simulink model "ASM_Traffic_V2X_Complete_Model_2"  (R2019a)
settings: Solver=ode1  StartTime=SIM.tstart.v  StopTime=Inf  FixedStep=SIM.StepSize.v  RelTol=1e-3
PostLoadFcn:
  | if any(exist('dsrtsu_mdlpostloadfcn', 'file') ~= 0), dsrtsu_mdlpostloadfcn('Execute', bdroot); end
  | try, asm_mdl_postloadfcn(bdroot, 'UpdateModel', 2200); catch, disp(lasterr); end,
undefined symbols (not defined in the file): _SensorPnts_1, _SensorPnts_13, _SensorPnts_17, _SensorPnts_21, _SensorPnts_25, _SensorPnts_29, _SensorPnts_33, _SensorPnts_37, _SensorPnts_41, _SensorPnts_45, _SensorPnts_49, _SensorPnts_5, _SensorPnts_53, _SensorPnts_57, _SensorPnts_9, _to_, CPT, G5A, ITS, MDL, rad, s_to_rpm, SIM
libraries: simulink x169, ASM_VehicleDynamics_lib x126, ASM_Traffic_lib x83, ASM_Utils_lib x49, mdbs x45, ASM_Environment_lib x17, dspindex x12, dsaV2xLibraryAux x10, dsmpblib x6, dsaV2xAsn1Library x4, dsaV2xLibrary x4, ASM_BrakeHydraulics_lib x4
(part 3 of 36)

== system ASM_Traffic_V2X_Complete_Model_2/IO/I//O_Subsystem/EgoCar_Command ==
  In1 : Inport
  In2 : Inport  Port=2
  Bus Creator : BusCreator  Inputs=4
  Bus Selector : BusSelector  OutputSignals=Simulated ECUs.DrivekitCAN.Drivekit.RX.PDUs.THROTTLE_COMMAND.throttle_pedal_command.ISignal Value.throttle_pedal_command Value,Simulated ECUs.DrivekitCAN.Drivekit.RX.PDUs.BRAKE_COMMAND.brake_pedal_command.ISignal Value.brake_pedal_command Value,Simulated ECUs.DrivekitCAN.Drivekit.RX.PDUs.STEERING_ANGLE_COMMAND.steering_angle_cmd_angle.ISignal Value.steering_angle_cmd_angle Value
  Data Type Conversion : DataTypeConversion  OutDataTypeStr=double
  Data Type Conversion1 : DataTypeConversion  OutDataTypeStr=double
  Data Type Conversion2 : DataTypeConversion  OutDataTypeStr=double
  Gain : Gain  Gain=100
  Gain1 : Gain  Gain=100
  Out1 : Outport
  wires:
  Gain1/1 -> Bus Creator/2
  Data Type Conversion1/1 -> Gain1/1
  Gain/1 -> Bus Creator/1
  Data Type Conversion/1 -> Gain/1
  Bus Creator/1 -> Out1/1
  In2/1 -> Bus Creator/4
  In1/1 -> Bus Selector/1
  Data Type Conversion2/1 -> Bus Creator/3
  Bus Selector/2 -> Data Type Conversion1/1  "<brake_pedal_command Value>"
  Bus Selector/3 -> Data Type Conversion2/1  "<steering_angle_cmd_angle Value>"
  Bus Selector/1 -> Data Type Conversion/1  "<throttle_pedal_command Value>"

== system ASM_Traffic_V2X_Complete_Model_2/IO/I//O_Subsystem/EgoCar_Data ==
  In1 : Inport
  Bus Creator : BusCreator  Inputs=4
  GPS : Subsystem
  Lane_Number : Subsystem
  Steering_Angle : Subsystem
  Wheel_Speed : Subsystem
  Out1 : Outport
  wires:
  Bus Creator/1 -> Out1/1
  GPS/1(Out1) -> Bus Creator/3
  Wheel_Speed/1(Out1) -> Bus Creator/2
  Steering_Angle/1(Out1) -> Bus Creator/1
  In1/1 -> Steering_Angle/1(In1), Wheel_Speed/1(In1), Lane_Number/1(In1), GPS/1(In1)
  Lane_Number/1(Out1) -> Bus Creator/4

== system ASM_Traffic_V2X_Complete_Model_2/IO/V2X_Subsystem/CAM-DENM_Message_Generation ==
  note: DENM
  note: CAM
  Input : Inport
  Bus Selector : BusSelector  OutputSignals=signal1,signal2,signal3,GenDENMData
  DENM : Subsystem
  Fellow_CAM_1 : Subsystem
  Fellow_CAM_2 : Subsystem
  Fellow_CAM_3 : Subsystem
  MSG_FREQ : DiscretePulseGenerator  PulseType=Time based  Period=0.5  PulseWidth=90
  Mux2 : Mux  Inputs=2
  Mux3 : Mux  Inputs=2
  Mux5 : Mux  Inputs=2
  OR : Logic  Operator=OR  Inputs=3  IconShape=distinctive  AllPortsSameDT=off  OutDataTypeStr=boolean
  Queue_CAM : Subsystem  TreatAsAtomicUnit=on
  Queue_CAM_DENM : Subsystem  TreatAsAtomicUnit=on
  Send_UDP : Subsystem  TreatAsAtomicUnit=on
  V2X_FREQ : DiscretePulseGenerator  PulseType=Time based  Period=0.5  PulseWidth=90
  wires:
  Queue_CAM_DENM/1(Data) -> Send_UDP/1(In1)
  V2X_FREQ/1 -> Send_UDP/Trigger
  MSG_FREQ/1 -> Queue_CAM_DENM/Trigger
  Queue_CAM_DENM/2(Byte) -> Send_UDP/2(Input)
  Mux5/1 -> Queue_CAM/1(Fellow_1)
  Fellow_CAM_2/1(Data) -> Mux3/1
  Fellow_CAM_2/2(Bytes) -> Mux3/2
  Fellow_CAM_1/1(Data) -> Mux5/1
  Fellow_CAM_1/2(Bytes) -> Mux5/2
  Mux2/1 -> Queue_CAM/3(Fellow_3)
  Fellow_CAM_3/1(Data) -> Mux2/1
  Fellow_CAM_3/2(Bytes) -> Mux2/2
  Mux3/1 -> Queue_CAM/2(Fellow_2)
  Fellow_CAM_1/3(Output_Enabler) -> OR/1, Queue_CAM/4(Enable_CAM1)
  Fellow_CAM_2/3(Output_Enabler) -> OR/2, Queue_CAM/5(Enable_CAM2)
  Fellow_CAM_3/3(Output_Enabler) -> OR/3, Queue_CAM/6(Enable_CAM3)
  OR/1 -> Queue_CAM_DENM/3(Enable_CAM), Queue_CAM/Enable
  Queue_CAM/1(OutputCAM) -> Queue_CAM_DENM/1(cam)
  DENM/1(denm_freq) -> Queue_CAM_DENM/4(Enable_DENM)
  DENM/2(denm) -> Queue_CAM_DENM/2(denm)
  Input/1 -> Bus Selector/1
  Bus Selector/1 -> Fellow_CAM_1/1(Input)  "<signal1>"
  Bus Selector/2 -> Fellow_CAM_2/1(Input)  "<signal2>"
  Bus Selector/3 -> Fellow_CAM_3/1(Input)  "<signal3>"
  Bus Selector/4 -> DENM/1("GENDENMData ")  "<GenDENMData>"

== system ASM_Traffic_V2X_Complete_Model_2/IO/V2X_Subsystem/Car_Data ==
  Fellow_Pos_info : Inport
  Bus Creator : BusCreator  Inputs=4
  EGOCAR_Position : Subsystem
  Fellow_ID_1 : Subsystem
  Fellow_ID_2 : Subsystem
  Fellow_ID_3 : Subsystem
  Subsystem : Subsystem
  Output : Outport
  wires:
  Bus Creator/1 -> Output/1
  Fellow_ID_3/1(Output) -> Bus Creator/3
  Fellow_ID_2/1(Output) -> Bus Creator/2
  Fellow_ID_1/1(Output) -> Bus Creator/1
  EGOCAR_Position/1(Output) -> Fellow_ID_1/1("EGO_Car_Position "), Subsystem/2(Input), Fellow_ID_3/1("EGO_Car_Position "), Fellow_ID_2/1("EGO_Car_Position ")
  Fellow_Pos_info/1 -> Fellow_ID_1/2(Input), Subsystem/3(Input1), Subsystem/1(In1), Fellow_ID_3/2(Input), Fellow_ID_2/2(Input), EGOCAR_Position/1(In1)
  Subsystem/1(Out1) -> Bus Creator/4

== system ASM_Traffic_V2X_Complete_Model_2/IO/V2X_Subsystem/Subsystem ==
  In1 : Inport
  AND : Logic  IconShape=distinctive  AllPortsSameDT=off  OutDataTypeStr=boolean
  AND1 : Logic  IconShape=distinctive  AllPortsSameDT=off  OutDataTypeStr=boolean
  AND_Display : Display
  Bus Selector : BusSelector  OutputSignals=Environment.Maneuver.ManeuverScheduler.Info.s_local[m],Environment.Maneuver.ManeuverScheduler.Info.t_local[s],Environment.Maneuver.ManeuverScheduler.Info.ManeuverTime[s],Environment.Driver.OutputSignals.Pos_BrakePedal[%],VehicleDynamics.VehicleMovement.Velocities.Vehicle.Linear.v_Vehicle_CoG[x;y;z][km|h].v_x_Vehicle_CoG[km|h],VehicleDynamics.VehicleMovement.Velocities.Vehicle.Linear.v_Total_Vehicle[km|h]
  Constant : Constant  Value=20
  Constant1 : Constant  Value=20
  Constant2 : Constant  Value=19.8
  Data Type Conversion{,1..4} (5 alike) : DataTypeConversion
  Relational Operator : RelationalOperator  Operator=<=  OutDataTypeStr=boolean  RndMeth=Simplest
  Relational Operator1 : RelationalOperator  OutDataTypeStr=boolean  RndMeth=Simplest
  Relational Operator2 : RelationalOperator  OutDataTypeStr=boolean  RndMeth=Simplest
  Subsystem : Subsystem
  driven_distance : Display
  manuever_time : Display
  pos_brake_pedal : Display
  speed_disp : Display
  start_of_spot_search : Display
  t_local : Display
  time_disp : Display
  v_ttotal_vehicle : Display
  v_x_vehicle : Display
  wires:
  In1/1 -> Bus Selector/1
  Bus Selector/1 -> Subsystem/1(In1), driven_distance/1  "<s_local[m]>"
  Bus Selector/2 -> t_local/1  "<t_local[s]>"
  Bus Selector/3 -> Relational Operator1/1, manuever_time/1  "<ManeuverTime[s]>"
  Bus Selector/4 -> pos_brake_pedal/1  "<Pos_BrakePedal[%]>"
  Bus Selector/5 -> Relational Operator2/1, Relational Operator/1, v_x_vehicle/1  "<v_x_Vehicle_CoG[km|h]>"
  Bus Selector/6 -> v_ttotal_vehicle/1  "<v_Total_Vehicle[km|h]>"
  Constant/1 -> Relational Operator/2
  Constant1/1 -> Relational Operator1/2
  Relational Operator1/1 -> Data Type Conversion/1
  Subsystem/1(Output) -> start_of_spot_search/1
  Constant2/1 -> Relational Operator2/2
  Relational Operator/1 -> Data Type Conversion1/1
  Relational Operator2/1 -> Data Type Conversion4/1
  AND1/1 -> Data Type Conversion2/1
  Data Type Conversion/1 -> time_disp/1, AND/1
  Data Type Conversion1/1 -> AND1/1, speed_disp/1
  Data Type Conversion2/1 -> AND/2
  AND/1 -> Data Type Conversion3/1
  Data Type Conversion3/1 -> Subsystem/Trigger, AND_Display/1
  Data Type Conversion4/1 -> AND1/2

== system ASM_Traffic_V2X_Complete_Model_2/MDL/Drivetrain/ASMSignalCollector ==
  BusCreator : BusCreator  Inputs=5
  tag scope: ASMBUS_Drivetrain=global
  wires:
  [ASMBUS_Drivetrain_FinalDriveAssembly] -> BusCreator/2
  [ASMBUS_Drivetrain_Test_Bench] -> BusCreator/5
  [ASMBUS_Drivetrain_Starter] -> BusCreator/4
  [ASMBUS_Drivetrain_CrankShaft] -> BusCreator/3
  [ASMBUS_Transmission] -> BusCreator/1
  BusCreator/1 -> [ASMBUS_Drivetrain]  "Drivetrain"

== system ASM_Traffic_V2X_Complete_Model_2/MDL/Drivetrain/Crankshaft ==
  Trq_TestBench[Nm] : Inport
  Trq_External[Nm] : Inport  Port=2
  Inertia_External[kgm2] : Inport  Port=3
  Reset[0|1] : Inport  Port=4
  Trq_Engine[Nm] : Inport  Port=5
  Trq_Fric_Clutch[Nm] : Inport  Port=6
  CRANK_SHAFT : ASM_VehicleDynamics_lib/Drivetrain/Crankshaft_and_Starter/CRANK_SHAFT  Tag=ASM_SUBCOMPONENT  Const_Inertia=MDL.Drivetrain.CrankShaft.Const_Inertia  Map_Trq_Mass=MDL.Drivetrain.CrankShaft.Map_Trq_Mass_Mod  Sw_Trq_Mass_Mode=MDL.Drivetrain.CrankShaft.Sw_Trq_Mass_Mode  StepSize=SIM.StepSize  ASMProperties=struct('Name','CRANK_SHAFT','Version','9.0','Library','ASM_VehicleDynamics_lib')  ASMInstanceName=crank_shaft  ASMInstanceID=1
  CrankAngle_Cyl[deg] : Constant  Value=0
  FROM_STABILIZATION_CRANK_SHAFT : ASM_VehicleDynamics_lib/Drivetrain/Stabilization/FROM_STABILIZATION  Tag=ASM_SUBCOMPONENT  Stabi_Block=CRANK_SHAFT  Stabi_Block_ID=1  ASMProperties=struct('Name','FROM_STABILIZATION','Version','1.0','Library','ASM_VehicleDynamics_lib')  ASMInstanceName=from_stabilization  ASMInstanceID=1
      settings: AttributesFormatString=Destination: CRANK_SHAFT_ID1
  TO_STABILIZATION_CRANK_SHAFT : ASM_VehicleDynamics_lib/Drivetrain/Stabilization/TO_STABILIZATION  Tag=ASM_SUBCOMPONENT  Stabi_Block=CRANK_SHAFT  Stabi_Block_ID=1  ASMProperties=struct('Name','TO_STABILIZATION','Version','1.0','Library','ASM_VehicleDynamics_lib')  ASMInstanceName=to_stabilization  ASMInstanceID=1
      settings: AttributesFormatString=Source: CRANK_SHAFT_ID1
  n_Engine_Init[rad|s] : Constant  Value=0
  n_Engine[rpm] : Outport
  n_Engine[rad|s] : Outport  Port=2
  tag scope: ASMBUS_Drivetrain_CrankShaft=global
  wires:
  FROM_STABILIZATION_CRANK_SHAFT/1 -> CRANK_SHAFT/9
  Trq_Fric_Clutch[Nm]/1 -> CRANK_SHAFT/3
  Inertia_External[kgm2]/1 -> CRANK_SHAFT/5
  Trq_TestBench[Nm]/1 -> CRANK_SHAFT/6
  Reset[0|1]/1 -> CRANK_SHAFT/4
  n_Engine_Init[rad|s]/1 -> CRANK_SHAFT/8
  CrankAngle_Cyl[deg]/1 -> CRANK_SHAFT/7
  Trq_Engine[Nm]/1 -> CRANK_SHAFT/2
  Trq_External[Nm]/1 -> CRANK_SHAFT/1
  CRANK_SHAFT/4 -> TO_STABILIZATION_CRANK_SHAFT/1
  CRANK_SHAFT/3 -> n_Engine[rad|s]/1
  CRANK_SHAFT/2 -> n_Engine[rpm]/1
  CRANK_SHAFT/1 -> [ASMBUS_Drivetrain_CrankShaft]

== system ASM_Traffic_V2X_Complete_Model_2/MDL/Drivetrain/DisableReset ==
  Reset_VehicleStates[0|1] : Inport
  MultiPortSwitch : MultiPortSwitch  DataPortOrder=Zero-based contiguous  Inputs=2  zeroidx=on  SaturateOnIntegerOverflow=on  InputSameDT=on
  NO_Reset : Constant  Value=0
  Reset[0|1] : Outport
  wires:
  Reset_VehicleStates[0|1]/1 -> MultiPortSwitch/3
  NO_Reset/1 -> MultiPortSwitch/2
  [TAG_Drivetrain_Sw_CrankShaft_Reset] -> MultiPortSwitch/1
  MultiPortSwitch/1 -> Reset[0|1]/1

== system ASM_Traffic_V2X_Complete_Model_2/MDL/Drivetrain/External Loads ==
  Inertia_TestBench[kgm2] : Inport
  Trq_Starter[Nm] : Inport  Port=2
  Inertia_Starter[kgm2] : Inport  Port=3
  Sw_AC[0|1] : Inport  Port=4
  Intertia_AC[kgm2] : Gain  Gain=0  SaturateOnIntegerOverflow=on  OutDataTypeStr=Inherit: Same as input  ParamDataTypeStr=Inherit: Same as input
  ManualLoadTorque : Subsystem
  Sum : Sum  Inputs=+++  SaturateOnIntegerOverflow=on
  Sum1 : Sum  Inputs=-+|  SaturateOnIntegerOverflow=on
  Trq_AC[Nm] : Gain  Gain=0  SaturateOnIntegerOverflow=on  OutDataTypeStr=Inherit: Same as input  ParamDataTypeStr=Inherit: Same as input
  Trq_External[Nm] : Outport
  Intertia_External[kgm2] : Outport  Port=2
  wires:
  Inertia_TestBench[kgm2]/1 -> Sum/1
  Intertia_AC[kgm2]/1 -> Sum/3
  Inertia_Starter[kgm2]/1 -> Sum/2
  ManualLoadTorque/1(Out) -> Trq_External[Nm]/1
  Trq_AC[Nm]/1 -> Sum1/1
  Sum1/1 -> ManualLoadTorque/1(In)
  Trq_Starter[Nm]/1 -> Sum1/2
  Sw_AC[0|1]/1 -> Trq_AC[Nm]/1, Intertia_AC[kgm2]/1
  Sum/1 -> Intertia_External[kgm2]/1

== system ASM_Traffic_V2X_Complete_Model_2/MDL/Drivetrain/Final_Drive_Assembly ==
  Inertia_Trm[kgm2] : Inport
  Trq_Out_Trm[Nm] : Inport  Port=2
  Reset[0|1] : Inport  Port=3
  omega_Wheel[FL,FR,RL,RR][rad|s] : Inport  Port=4
  ASMSignalCollector : Subsystem
  Differentials : Subsystem
  FF4WD_Parts : Subsystem
  GotoTagVisibility_CentralDifferential : GotoTagVisibility  GotoTag=ASMBUS_Drivetrain_CentralDifferential
  GotoTagVisibility_Clutch_4WD : GotoTagVisibility  GotoTag=ASMBUS_Drivetrain_Clutch_4WD
  GotoTagVisibility_FrontDifferential : GotoTagVisibility  GotoTag=ASMBUS_Drivetrain_FrontDifferential
  GotoTagVisibility_RearDifferential : GotoTagVisibility  GotoTag=ASMBUS_Drivetrain_RearDifferential
  GotoTagVisibility_Shaft_CF : GotoTagVisibility  GotoTag=ASMBUS_Drivetrain_Shaft_CF
  GotoTagVisibility_Shaft_CR : GotoTagVisibility  GotoTag=ASMBUS_Drivetrain_Shaft_CR
  GotoTagVisibility_Shaft_FL : GotoTagVisibility  GotoTag=ASMBUS_Drivetrain_Shaft_FL
  GotoTagVisibility_Shaft_FR : GotoTagVisibility  GotoTag=ASMBUS_Drivetrain_Shaft_FR
  GotoTagVisibility_Shaft_RL : GotoTagVisibility  GotoTag=ASMBUS_Drivetrain_Shaft_RL
  GotoTagVisibility_Shaft_RR : GotoTagVisibility  GotoTag=ASMBUS_Drivetrain_Shaft_RR
  GotoTagVisibility_Shaft_TGCL4WD : GotoTagVisibility  GotoTag=ASMBUS_Drivetrain_Shaft_TGCL4WD
  GotoTagVisibility_Transfer_Gearbox : GotoTagVisibility  GotoTag=ASMBUS_Drivetrain_Transfer_Gearbox
  STABILIZATION : Subsystem
  Shafts : Subsystem
  SignalSelection : Subsystem
  omega_In_Diff[rad|s] : Outport
  Trq_Shaft[FL,FR,RL,RR][Nm] : Outport  Port=2
  wires:
  Reset[0|1]/1 -> FF4WD_Parts/3(Reset[0|1]), Shafts/10(Reset[0|1]), Differentials/15(Reset[0|1])
  FF4WD_Parts/1(Inertia_Out_Clutch4WD[kgm2]) -> SignalSelection/6(Inertia_Out_Clutch4WD[kgm2])
  FF4WD_Parts/2(Trq_Lock_Clutch4WD[Nm]) -> SignalSelection/5(Trq_Lock_Clutch4WD[Nm])
  FF4WD_Parts/3(Inertia_In_TransferGearbox[kgm2]) -> SignalSelection/4(Inertia_In_TransferGearbox[kgm2])
  FF4WD_Parts/4(Trq_In_TransferGearbox[Nm]) -> SignalSelection/3(Trq_In_TransferGearbox[Nm])
  SignalSelection/6(Inertia_External_InputShaft_RearDiff[kgm2]) -> Differentials/8(Inertia_External_InputShaft_RearDiff[kgm2])
  SignalSelection/5(Trq_In_RearDiff[Nm]) -> Differentials/7(Trq_In_RearDiff[Nm])
  SignalSelection/4(Inertia_Ext_Cage_FrontDiff[kgm2]) -> Differentials/6(Inertia_Ext_Cage_FrontDiff[kgm2])
  SignalSelection/3(Trq_Ext_Cage_FrontDiff[Nm]) -> Differentials/5(Trq_Ext_Cage_FrontDiff[Nm])
  SignalSelection/2(Inertia_External_InputShaft_FrontDiff[kgm2]) -> Differentials/4(Inertia_External_InputShaft_FrontDiff[kgm2])
  SignalSelection/1(Trq_In_FrontDiff[Nm]) -> Differentials/3(Trq_In_FrontDiff[Nm])
  Differentials/2(omega_Cage_FrontDiff[rad|s]) -> FF4WD_Parts/5(omega_Cage_FrontDiff[rad|s])
  Differentials/3(omega_In_RearDiff[rad|s]) -> FF4WD_Parts/4(omega_In_RearDiff[rad|s]), Shafts/8(omega_In_RearDiff[rad|s])
  Differentials/4(omega_In_FrontDiff[rad|s]) -> Shafts/7(omega_In_FrontDiff[rad|s])
  Differentials/6(omega_Out_Rear_CentralDiff[rad|s]) -> Shafts/5(omega_Out_Rear_CentralDiff[rad|s])
  Differentials/5(omega_Out_Front_CentralDiff[rad|s]) -> Shafts/6(omega_Out_Front_CentralDiff[rad|s])
  Shafts/4(Trq_CR_Shaft[Nm]) -> Differentials/11(Trq_CR_Shaft[Nm]), SignalSelection/8(Trq_CR_Shaft[Nm])
  Shafts/3(Trq_CF_Shaft[Nm]) -> Differentials/12(Trq_CF_Shaft[Nm]), SignalSelection/7(Trq_CF_Shaft[Nm])
  omega_Wheel[FL,FR,RL,RR][rad|s]/1 -> Shafts/9(omega_Wheel[FL,FR,RL,RR][rad|s])
  Shafts/7(Trq_Shaft[FL,FR,RL,RR][Nm]) -> Trq_Shaft[FL,FR,RL,RR][Nm]/1
  Differentials/10(omega_Out_Right_RearDiff[rad|s]) -> Shafts/1(omega_Out_Right_RearDiff[rad|s])
  Differentials/9(omega_Out_Left_RearDiff[rad|s]) -> Shafts/2(omega_Out_Left_RearDiff[rad|s])
  Differentials/8(omega_Out_Right_FrontDiff[rad|s]) -> Shafts/3(omega_Out_Right_FrontDiff[rad|s])
  Differentials/7(omega_Out_Left_FrontDiff[rad|s]) -> Shafts/4(omega_Out_Left_FrontDiff[rad|s])
  Differentials/1(omega_In_Diff[rad|s]) -> omega_In_Diff[rad|s]/1
  Shafts/5(Trq_RR_Shaft[Nm]) -> FF4WD_Parts/2(Trq_RR_Shaft[Nm]), Differentials/10(Trq_RR_Shaft[Nm])
  Shafts/6(Trq_RL_Shaft[Nm]) -> FF4WD_Parts/1(Trq_RL_Shaft[Nm]), Differentials/9(Trq_RL_Shaft[Nm])
  Shafts/1(Trq_FR_Shaft[Nm]) -> Differentials/14(Trq_FR_Shaft[Nm])
  Shafts/2(Trq_FL_Shaft[Nm]) -> Differentials/13(Trq_FL_Shaft[Nm])
  Trq_Out_Trm[Nm]/1 -> Differentials/2(Trq_Out_Trm[Nm]), SignalSelection/2(Trq_Out_Trm[Nm])
  Inertia_Trm[kgm2]/1 -> Differentials/1(Inertia_Trm[kgm2]), SignalSelection/1(Inertia_Trm[kgm2])

== system ASM_Traffic_V2X_Complete_Model_2/MDL/Drivetrain/OpenCrankshaftDemos ==

== system ASM_Traffic_V2X_Complete_Model_2/MDL/Drivetrain/OpenFinalDriveAssemblyDemos ==

== system ASM_Traffic_V2X_Complete_Model_2/MDL/Drivetrain/OpenTransmissionSystemDemos ==

== system ASM_Traffic_V2X_Complete_Model_2/MDL/Drivetrain/Transmission ==
  Trq_Engine[Nm] : Inport
  n_Engine[rad|s] : Inport  Port=2
  Ctrl_Lockup_Clutch[%] : Inport  Port=3
  Gear_AT[] : Inport  Port=4
  Pos_ClutchPedal_MT[%] : Inport  Port=5
  Gear_MT[] : Inport  Port=6
  SW_TrmMode[1Manual|2Automatic] : Inport  Port=7
  Reset[0|1] : Inport  Port=8
  omega_In_Diff[rad|s] : Inport  Port=9
  ASMSignalCollector : Subsystem
  AutomaticActive : simulink/Logic and Bit Operations/Compare To Constant  relop===  const=2  OutDataTypeStr=boolean
  AutomaticTransmission : Subsystem  TreatAsAtomicUnit=on
  FROM_STABILIZATION_CLUTCH : ASM_VehicleDynamics_lib/Drivetrain/Stabilization/FROM_STABILIZATION  Tag=ASM_SUBCOMPONENT  Stabi_Block=CLUTCH  Stabi_Block_ID=1  ASMProperties=struct('Name','FROM_STABILIZATION','Version','1.0','Library','ASM_VehicleDynamics_lib')  ASMInstanceName=from_stabilization  ASMInstanceID=1
      settings: AttributesFormatString=Destination: CLUTCH_ID1
  ManualActive : simulink/Logic and Bit Operations/Compare To Constant  relop===  const=1  OutDataTypeStr=boolean
  ManualTransmission : Subsystem  TreatAsAtomicUnit=on
  Multiport Switch{,1..5} (6 alike) : MultiPortSwitch  Inputs=2  SaturateOnIntegerOverflow=on
  Sat_TrmMode : Saturate  UpperLimit=2  LowerLimit=1
  TO_STABILIZATION_CLUTCH : ASM_VehicleDynamics_lib/Drivetrain/Stabilization/TO_STABILIZATION  Tag=ASM_SUBCOMPONENT  Stabi_Block=CLUTCH  Stabi_Block_ID=1  ASMProperties=struct('Name','TO_STABILIZATION','Version','1.0','Library','ASM_VehicleDynamics_lib')  ASMInstanceName=to_stabilization  ASMInstanceID=1
      settings: AttributesFormatString=Source: CLUTCH_ID1
  TO_STABILIZATION_GEARBOX : ASM_VehicleDynamics_lib/Drivetrain/Stabilization/TO_STABILIZATION  Tag=ASM_SUBCOMPONENT  Stabi_Block=GEARBOX  Stabi_Block_ID=1  ASMProperties=struct('Name','TO_STABILIZATION','Version','1.0','Library','ASM_VehicleDynamics_lib')  ASMInstanceName=to_stabilization  ASMInstanceID=1
      settings: AttributesFormatString=Source: GEARBOX_ID1
  TO_STABILIZATION_TORQUE_CONVERTER : ASM_VehicleDynamics_lib/Drivetrain/Stabilization/TO_STABILIZATION  Tag=ASM_SUBCOMPONENT  Stabi_Block=TORQUE_CONVERTER  Stabi_Block_ID=1  ASMProperties=struct('Name','TO_STABILIZATION','Version','1.0','Library','ASM_VehicleDynamics_lib')  ASMInstanceName=to_stabilization  ASMInstanceID=1
      settings: AttributesFormatString=Source: TORQUE_CONVERTER_ID1
  Trq_Fric[Nm] : Outport
  Inertia_Out_Trm[kgm2] : Outport  Port=2
  Trq_Out_Trm[Nm] : Outport  Port=3
  tag scope: ASMBUS_Drivetrain_AutomaticTransmission=global, ASMBUS_Drivetrain_ManualTransmission=global
  wires:
  Multiport Switch5/1 -> TO_STABILIZATION_CLUTCH/1
  Multiport Switch4/1 -> TO_STABILIZATION_GEARBOX/1
  ManualTransmission/5(TO_STABILIZATION_GEARBOX) -> Multiport Switch4/2
  AutomaticTransmission/6(TO_STABILIZATION_CLUTCH) -> Multiport Switch5/3
  AutomaticTransmission/7(TO_STABILIZATION_TORQUE_CONVERTER) -> TO_STABILIZATION_TORQUE_CONVERTER/1
  Sat_TrmMode/1 -> Multiport Switch/1, Multiport Switch1/1, Multiport Switch2/1, Multiport Switch4/1, Multiport Switch5/1, ASMSignalCollector/1(SW_TrmMode[]), Multiport Switch3/1, ManualActive/1, AutomaticActive/1
  Reset[0|1]/1 -> AutomaticTransmission/7(Reset[0|1]), ManualTransmission/7(Reset[0|1])
  AutomaticTransmission/5(TO_STABILIZATION_GEARBOX) -> Multiport Switch4/3
  AutomaticTransmission/4(Inertia_Out_Trm[kgm2]) -> Multiport Switch2/3
  AutomaticTransmission/3(Trq_Out_Trm[Nm]) -> Multiport Switch1/3
  AutomaticTransmission/2(Trq_In_Converter[Nm]) -> Multiport Switch/3
  ManualTransmission/6(TO_STABILIZATION_CLUTCH) -> Multiport Switch5/2
  Multiport Switch1/1 -> Trq_Out_Trm[Nm]/1
  Multiport Switch/1 -> Trq_Fric[Nm]/1
  Multiport Switch2/1 -> Inertia_Out_Trm[kgm2]/1
  ManualTransmission/2(Trq_Fric[Nm]) -> Multiport Switch/2
  ManualTransmission/3(Trq_Out_Trm[Nm]) -> Multiport Switch1/2
  ManualTransmission/4(Inertia_Out_Trm[kgm2]) -> Multiport Switch2/2
  SW_TrmMode[1Manual|2Automatic]/1 -> Sat_TrmMode/1
  Pos_ClutchPedal_MT[%]/1 -> ManualTransmission/1(Pos_Clutch[%])
  Gear_MT[]/1 -> ManualTransmission/2(Gear[]), Multiport Switch3/2
  n_Engine[rad|s]/1 -> AutomaticTransmission/3(n_Engine[rad|s]), ManualTransmission/3(n_Engine[rad|s])
  Trq_Engine[Nm]/1 -> AutomaticTransmission/4(Trq_Engine[Nm]), ManualTransmission/4(Trq_Engine[Nm])
  omega_In_Diff[rad|s]/1 -> AutomaticTransmission/5(omega_In_Diff[rad|s]), ManualTransmission/5(omega_In_Diff[rad|s])
  AutomaticActive/1 -> AutomaticTransmission/Enable
  FROM_STABILIZATION_CLUTCH/1 -> AutomaticTransmission/6(FROM_STABILIZATION_CLUTCH), ManualTransmission/6(FROM_STABILIZATION_CLUTCH)
  ManualActive/1 -> ManualTransmission/Enable
  Ctrl_Lockup_Clutch[%]/1 -> AutomaticTransmission/1(Ctrl_Lockup_Clutch[%])
  Gear_AT[]/1 -> AutomaticTransmission/2(Gear[]), Multiport Switch3/3
  Multiport Switch3/1 -> ASMSignalCollector/2(Gear[])
  ManualTransmission/1(ASMSignalBus) -> [ASMBUS_Drivetrain_ManualTransmission]
  AutomaticTransmission/1(ASMSignalBus) -> [ASMBUS_Drivetrain_AutomaticTransmission]

== system ASM_Traffic_V2X_Complete_Model_2/MDL/Engine/ASMSignalCollector ==
  BusCreator : BusCreator  Inputs=2
  tag scope: ASMBUS_EngineBasic=global
  wires:
  [ASMBUS_EngineBasic_FuelConsumption] -> BusCreator/2
  BusCreator/1 -> [ASMBUS_EngineBasic]  "BasicEngine"
  [ASMBUS_EngineBasic_EngineBasic] -> BusCreator/1

== system ASM_Traffic_V2X_Complete_Model_2/MDL/Environment/ASMSignalCollector ==
  Bus Creator : BusCreator  Inputs=4
  tag scope: ASMBUS_Environment=global
  wires:
  [ASMBUS_Environment_Driver] -> Bus Creator/1
  Bus Creator/1 -> [ASMBUS_Environment]  "Environment"
  [ASMBUS_Environment_Road] -> Bus Creator/2
  [ASMBUS_Environment_Maneuver] -> Bus Creator/3
  [ASMBUS_Environment_Traffic] -> Bus Creator/4

== system ASM_Traffic_V2X_Complete_Model_2/MDL/Environment/Driver ==
  note: eGO Car Inputs from ControlPC via CAN Bus
  Road_Signals : Inport
  Maneuver_Signals : Inport  Port=2
  VehicleDynamics_Signals : Inport  Port=3
  Drivetrain_Signals : Inport  Port=4
  SoftECU_Engine_Signals : Inport  Port=5
  Input : Inport  Port=6
  ASMSignalCollector : Subsystem
  Bus Selector : BusSelector  OutputSignals=VehicleMovement.Velocities.v_x_Vehicle[km|h]
  Bus Selector1 : BusSelector  OutputSignals=VehicleMovement.Velocities.v_x_Vehicle[km|h]
  COMMON_DRIVER_PARAMETERS : ASM_Environment_lib/Environment/Driver/COMMON_DRIVER_PARAMETERS  Tag=ASM_SUBCOMPONENT  Const_Angle_Max_SteeringWheel=MDL.Environment.Driver.Const_Angle_Max_SteeringWheel  ASMProperties=struct('Name','COMMON_DRIVER_PARAMETERS','Version','3.0','Library','ASM_Environment_lib')  ASMInstanceName=common_driver_parameters  ASMInstanceID=1
  LateralController : Subsystem
  LongitudinalController : Subsystem
  Mux : Mux  Inputs=2
  ReferenceVelocity : Subsystem
  SignalSelection : Subsystem
  Source_of_eGoCAR_Control_Conditions : Subsystem
      mask Display: image('steeringwheel.jpg');
  SteeringWheelAngle_Control : Subsystem
  Terminator4 : Terminator
  Driver_Signals : Outport
  s_Preview[m] : Outport  Port=2
  wires:
  LongitudinalController/2(Pos_BrakePedal[%]) -> Source_of_eGoCAR_Control_Conditions/3(Break_Input_SIM)
  LongitudinalController/6(t_Preview_vRef[s]) -> SignalSelection/7(t_Preview_vRef[s])
  ReferenceVelocity/2(v_Vehicle_Ref_Preview[m|s]) -> LongitudinalController/6(v_Vehicle_Ref_Preview[m|s])
  SignalSelection/1(Driver_Signals) -> Driver_Signals/1
  SoftECU_Engine_Signals/1 -> LongitudinalController/3(SoftECU_Engine_Signals)
  LongitudinalController/5(SelectorLever[-3T|-2P|-1R|0N|1D]) -> SignalSelection/6(SelectorLever_Driver[-3T|-2P|-1R|0N|1D])
  Drivetrain_Signals/1 -> LongitudinalController/2(Drivetrain_Signals)
  Road_Signals/1 -> LateralController/3(Road_Signals), ReferenceVelocity/3(Road_Signals)
  VehicleDynamics_Signals/1 -> Bus Selector1/1, Bus Selector/1, LateralController/2(VehicleDynamics_Signals), ReferenceVelocity/2(VehicleDynamics_Signals), LongitudinalController/4(VehicleDynamics_Signals)
  Maneuver_Signals/1 -> LateralController/1(Maneuver_Signals), ReferenceVelocity/1(Maneuver_Signals), LongitudinalController/1(Maneuver_Signals), SignalSelection/1(Maneuver_Signals)
  LongitudinalController/4(Gear[]) -> SignalSelection/5(Gear[])
  LongitudinalController/3(Pos_ClutchPedal[%]) -> SignalSelection/4(Pos_ClutchPedal[%])
  ReferenceVelocity/3(s_Preview_vRef[m]) -> Mux/1
  ReferenceVelocity/1(v_Vehicle_Ref[m|s]) -> LongitudinalController/5(v_Vehicle_Ref[m|s])
  LateralController/1(s_Preview_LatCtrl[m]) -> Mux/2
  Mux/1 -> s_Preview[m]/1
  Bus Selector1/1 -> SteeringWheelAngle_Control/2(Speed)  "<v_x_Vehicle[km|h]>"
  LongitudinalController/1(Pos_AccPedal[%]) -> Source_of_eGoCAR_Control_Conditions/2(Throttle_Input_SIM)
  SteeringWheelAngle_Control/1(SteerWheelAngle) -> Terminator4/1
  Input/1 -> Source_of_eGoCAR_Control_Conditions/1(In1)
  LateralController/2(Angle_SteeringWheel_LatCtrl[deg]) -> Source_of_eGoCAR_Control_Conditions/4(Steering_Input_SIM), SteeringWheelAngle_Control/1(SteerWheelAngle_from_Sim)
  Source_of_eGoCAR_Control_Conditions/1(Throttle) -> SignalSelection/2(Pos_AccPedal[%])
  Source_of_eGoCAR_Control_Conditions/2(Break) -> SignalSelection/3(Pos_BrakePedal[%])
  Source_of_eGoCAR_Control_Conditions/3(Steering) -> SignalSelection/8(Angle_SteeringWheel[deg])
  Bus Selector/1 -> Source_of_eGoCAR_Control_Conditions/5(eGOCAR_Speed_kmh)  "<v_x_Vehicle[km|h]>"

== system ASM_Traffic_V2X_Complete_Model_2/MDL/Environment/EnvironmentInterface_In ==
  Vehicle_Signals : Inport
  Bus Creator : BusCreator  Inputs=3
  Bus Selector1 : BusSelector  OutputSignals=VehicleDynamics.Steering,VehicleDynamics.Tire,VehicleDynamics.VehicleMovement,VehicleDynamics.Aerodynamics,Drivetrain,SoftECU
  Drivetrain : Subsystem
  SoftECU_Engine : Subsystem
  Steering : Subsystem
  Tire : Subsystem
  VehicleMovement : Subsystem
  VehicleDynamics_Signals : Outport
  Drivetrain_Signals : Outport  Port=2
  SoftECU_Signals : Outport  Port=3
  wires:
  Bus Selector1/4 -> VehicleMovement/2(Aerodynamics)  "<Aerodynamics>"
  SoftECU_Engine/1(SoftECU_Signals) -> SoftECU_Signals/1
  Bus Selector1/6 -> SoftECU_Engine/1(SoftECU)  "<SoftECU>"
  Drivetrain/1(Drivetrain_Signals) -> Drivetrain_Signals/1
  Vehicle_Signals/1 -> Bus Selector1/1
  Bus Creator/1 -> VehicleDynamics_Signals/1
  Bus Selector1/1 -> Steering/1(Steering)  "<Steering>"
  Bus Selector1/2 -> Tire/1(Tire)  "<Tire>"
  Bus Selector1/3 -> VehicleMovement/1(VehicleMovement)  "<VehicleMovement>"
  Steering/1(Steering_Signals) -> Bus Creator/1
  Tire/1(Tire_Signals) -> Bus Creator/2
  VehicleMovement/1(VehicleMovement_Signals) -> Bus Creator/3
  Bus Selector1/5 -> Drivetrain/1(Drivetrain)  "<Drivetrain>"

== system ASM_Traffic_V2X_Complete_Model_2/MDL/Environment/Maneuver ==
  Road_Signals : Inport
  VehicleDynamics_Signals : Inport  Port=2
  Driver_Signals : Inport  Port=3
  Traffic_Signals : Inport  Port=4
  SoftECU_Signals : Inport  Port=5
  ASMSignalCollector : Subsystem
  AvoidAlgLoop{,1..9} (10 alike) : Memory
  Bus Creator1 : BusCreator  Inputs=13
  Bus Selector : BusSelector  OutputSignals=Road_Info.RoadState[],Road_ASMVeh.s_Veh_Road[m],Road_ASMVeh.s_Total_Veh_Road[m],Road_ASMVeh.s_Veh_Road_Trj[m],Road_Info.Dist_Response_Maneuver.Distance_xy[m]
  Bus Selector1 : BusSelector  OutputSignals=VehicleMovement.Positions.s_Vehicle[m],VehicleMovement.Velocities.v_x_Vehicle[km|h],VehicleMovement.Accelerations.a_y_Vehicle_CoG[m|s2],Tire.r_Dyn_Tire_Mean[m]
  Bus Selector2 : BusSelector  OutputSignals=v_Vehicle_Init[km|h]
  Bus Selector3 : BusSelector  OutputSignals=Keep_VehiclePosition[0|1]
  Bus Selector4 : BusSelector  OutputSignals=ManeuverState[]
  Bus Selector5 : BusSelector  OutputSignals=ManeuverState[]
  Bus Selector6 : BusSelector  OutputSignals=t_Preview_vRef[s]
  Bus Selector7 : BusSelector  OutputSignals=FellowMovement.Dist_Refline_Response[m]
  Customize_UserSignals : Subsystem
  Demux3 : Demux
  ExternalSegmentEnd : Subsystem
  ExternalUserData : Subsystem
  LastValues : Subsystem
  LogOp_Or_ExtReset : Logic  Operator=OR  AllPortsSameDT=off
  MANEUVER_SCHEDULER : ASM_Environment_lib/Environment/Maneuver/MANEUVER_SCHEDULER  Tag=ASM_SUBCOMPONENT  Maneuver_ModelDesk=MDL.Environment.Maneuver.Maneuver_ModelDesk  Maneuver_2=MDL.Environment.Maneuver.Maneuver_2  Maneuver_3=MDL.Environment.Maneuver.Maneuver_3  Maneuver_4=MDL.Environment.Maneuver.Maneuver_4  Maneuver_5=MDL.Environment.Maneuver.Maneuver_5  Maneuver_6=MDL.Environment.Maneuver.Maneuver_6  ASMProperties=struct('Name','MANEUVER_SCHEDULER','Version','21.0','Library','ASM_Environment_lib')  ASMInstanceName=maneuver_scheduler  ASMInstanceID=1
  MANEUVER_STATE : ASM_Utils_lib/ModelDeskInterface/ManeuverControl/MANEUVER_STATE  Tag=ASM_SUBCOMPONENT  ASMProperties=struct('Name','MANEUVER_STATE','Version','1.0','Library','ASM_Utils_lib')  ASMInstanceName=maneuver_state  ASMInstanceID=1
  MODEL_DESK_WRITE_ACCESS : ASM_Utils_lib/ModelDeskInterface/MODEL_DESK_WRITE_ACCESS  Tag=ASM_SUBCOMPONENT  ASMProperties=struct('Name','MODEL_DESK_WRITE_ACCESS','Version','1.0','Library','ASM_Utils_lib')  ModelDesk_WriteAccess=MDL.Environment.ModelDesk_WriteAccess  ASMInstanceName=model_desk_write_access  ASMInstanceID=1
  ParkingBrake : Subsystem
  ReplaceBrake : Subsystem
  ReplaceSelectorLever_Mode : Subsystem
  Reset _IfModeSwitched : Subsystem
  SimulationControl : Subsystem
  StartButton : Subsystem
  StartButton_ManSched[0Off|1On] : Constant  Value=0
  Testbench : Subsystem
  TipShift : Subsystem
  UnitConversion : ASM_Utils_lib/UnitConversion/UnitConversion  Selection=km/h_to_m/s
  VehicleInitStates : Subsystem
  Maneuver_Signals : Outport
  tag scope: ASMBUS_Environment_ManeuverScheduler=global, ASMBUS_Environment_Mnvr_UserSignalsCustomized=global
  wires:
  AvoidAlgLoop9/1 -> MANEUVER_SCHEDULER/13
  Bus Selector/4 -> AvoidAlgLoop9/1  "<s_Veh_Road_Trj[m]>"
  Bus Selector7/1 -> MANEUVER_SCHEDULER/15  "<Dist_Refline_Response[m]>"
  StartButton_ManSched[0Off|1On]/1 -> StartButton/1(StartButton_ManSched[0Off|1On])
  [TAG_StartButton_Signals] -> StartButton/2(StartButton_Signals_)
  ReplaceSelectorLever_Mode/1(ModeSignals) -> Bus Creator1/3
  MANEUVER_SCHEDULER/4 -> ReplaceSelectorLever_Mode/1(ModeSignals_In)
  [TAG_SW_TipShift] -> TipShift/1(SW_TipTronic[-1Down|0Off|1Up])
  AvoidAlgLoop8/1 -> MANEUVER_SCHEDULER/23
  Bus Selector6/1 -> AvoidAlgLoop8/1  "<t_Preview_vRef[s]>"
  Bus Selector5/1 -> MANEUVER_STATE/1  "<ManeuverState[]>"
  SoftECU_Signals/1 -> ExternalSegmentEnd/4(SoftECU_Signals)
  Bus Selector2/1 -> VehicleInitStates/3(v_Vehicle_Init_Mnv[km|h])  "<v_Vehicle_Init[km|h]>"
  Bus Selector/5 -> AvoidAlgLoop7/1  "<Distance_xy[m]>"
  AvoidAlgLoop7/1 -> MANEUVER_SCHEDULER/14
  Bus Creator1/1 -> Maneuver_Signals/1  "Maneuver"
  [TAG_Sw_ManeuverControl] -> Demux3/1
  MANEUVER_SCHEDULER/1 -> [ASMBUS_Environment_ManeuverScheduler]
  UnitConversion/1 -> AvoidAlgLoop1/1
  Bus Selector1/2 -> UnitConversion/1  "<v_x_Vehicle[km|h]>"
  Bus Selector1/1 -> AvoidAlgLoop2/1  "<s_Vehicle[m]>"
  Bus Selector1/3 -> AvoidAlgLoop/1  "<a_y_Vehicle_CoG[m|s2]>"
  Bus Selector/2 -> AvoidAlgLoop3/1  "<s_Veh_Road[m]>"
  Bus Selector/1 -> AvoidAlgLoop4/1  "<RoadState[]>"
  MODEL_DESK_WRITE_ACCESS/1 -> MANEUVER_SCHEDULER/8
  [TAG_Sw_ManeuverSelect] -> MANEUVER_SCHEDULER/1
  MANEUVER_SCHEDULER/2 -> Bus Creator1/1, Bus Selector3/1
  MANEUVER_SCHEDULER/3 -> Bus Selector2/1, Bus Creator1/2
  MANEUVER_SCHEDULER/6 -> Bus Creator1/5
  Bus Selector/3 -> AvoidAlgLoop5/1  "<s_Total_Veh_Road[m]>"
  [TAG_Sw_Transmission_Mode] -> Reset _IfModeSwitched/2(TrmMode)
  [TAG_Sw_Tire_Model] -> Reset _IfModeSwitched/3(TireMode)
  Demux3/4 -> LogOp_Or_ExtReset/1
  Reset _IfModeSwitched/1(Reset_IfModeSwitched) -> LogOp_Or_ExtReset/2
  Driver_Signals/1 -> Bus Selector6/1, LastValues/2(Driver_Signals)
  Road_Signals/1 -> Bus Selector/1, ExternalSegmentEnd/1(Road_Signals), LastValues/3(Road_Signals)
  [TAG_Sw_Drivetrain_Mode] -> Reset _IfModeSwitched/1(DrvTrnMode)
  MANEUVER_SCHEDULER/5 -> ReplaceBrake/1(RefSignals_In), LastValues/4(Maneuver_RefSignals)
  ReplaceBrake/1(RefSignals) -> Bus Creator1/4
  Customize_UserSignals/2(UserSignals_Customized) -> ExternalSegmentEnd/5(UserSignals_Customized), Bus Creator1/8
  Customize_UserSignals/1(ASMSignalBus) -> [ASMBUS_Environment_Mnvr_UserSignalsCustomized]
  [TAG_SW_ParkingBrake] -> ParkingBrake/1(Sw_ParkingBrake[0Off|1On])
  [TAG_n_Engine_Set] -> Testbench/2(n_Engine_Set[rpm])
  [TAG_SW_Testbench] -> Testbench/1(SW_Testbench[0Off|1On])
  Bus Selector3/1 -> VehicleInitStates/1(Keep_VehiclePosition[0|1])  "<Keep_VehiclePosition[0|1]>"
  [TAG_Vehicle_Init] -> VehicleInitStates/4(VehicleInitStates_External)
  Bus Selector4/1 -> VehicleInitStates/2(ManeuverState[])  "<ManeuverState[]>"
  Traffic_Signals/1 -> ExternalSegmentEnd/3(Traffic_Signals), Bus Selector7/1
  Demux3/1 -> MANEUVER_SCHEDULER/3
  Demux3/2 -> MANEUVER_SCHEDULER/4
  Demux3/3 -> MANEUVER_SCHEDULER/5
  LogOp_Or_ExtReset/1 -> MANEUVER_SCHEDULER/6
  [TAG_Const_PedalsManualDriving] -> MANEUVER_SCHEDULER/20
  Bus Selector1/4 -> AvoidAlgLoop6/1  "<r_Dyn_Tire_Mean[m]>"
  [TAG_Sw_ManeuverSettings] -> MANEUVER_SCHEDULER/2
  LastValues/1(LastValues) -> MANEUVER_SCHEDULER/9
  AvoidAlgLoop4/1 -> MANEUVER_SCHEDULER/10
  AvoidAlgLoop3/1 -> MANEUVER_SCHEDULER/11
  AvoidAlgLoop5/1 -> MANEUVER_SCHEDULER/12
  AvoidAlgLoop2/1 -> MANEUVER_SCHEDULER/16
  AvoidAlgLoop1/1 -> MANEUVER_SCHEDULER/17
  AvoidAlgLoop/1 -> MANEUVER_SCHEDULER/18
  AvoidAlgLoop6/1 -> MANEUVER_SCHEDULER/19
  ExternalUserData/1(External_ReferenceSignals) -> MANEUVER_SCHEDULER/21
  ExternalSegmentEnd/1(External_SegmentEnd[0|1]) -> MANEUVER_SCHEDULER/22
  SimulationControl/1(Keep_VehiclePosition[0|1]) -> MANEUVER_SCHEDULER/7
  VehicleDynamics_Signals/1 -> SimulationControl/1(VehicleDynamics_Signals), Bus Selector1/1, ExternalSegmentEnd/2(VehicleDynamics_Signals), LastValues/1(VehicleDynamics_Signals)
  MANEUVER_SCHEDULER/8 -> Customize_UserSignals/1(UserSignals_In), Bus Creator1/7
  MANEUVER_SCHEDULER/7 -> ReplaceBrake/2(Info), Bus Selector4/1, Bus Selector5/1, Bus Creator1/6
  VehicleInitStates/1(VehicleInitStates) -> Bus Creator1/9
  TipShift/1(TipShiftSignals) -> Bus Creator1/10
  StartButton/1(StartButton_Signals) -> Bus Creator1/11
  ParkingBrake/1(ParkingBrakeSignals) -> Bus Creator1/12
  Testbench/1(Testbench) -> Bus Creator1/13

== system ASM_Traffic_V2X_Complete_Model_2/MDL/Environment/Road ==
  s_Preview[m] : Inport
  Maneuver_Signals : Inport  Port=2
  VehicleDynamics_Signals : Inport  Port=3
  Traffic_Signals : Inport  Port=4
  AMBIENT : ASM_Environment_lib/Environment/Road/AMBIENT  Tag=ASM_SUBCOMPONENT  Const_temperature=MDL.Environment.Ambient.Const_T  Const_pressure=MDL.Environment.Ambient.Const_p  ASMProperties=struct('Name','AMBIENT','Version','2.0','Library','ASM_Environment_lib')  ASMInstanceName=ambient  ASMInstanceID=1
  ASMSignalCollector : Subsystem
  BASIC_ROADS : ASM_Environment_lib/Environment/Road/BASIC_ROADS  Tag=ASM_SUBCOMPONENT  StepSize=SIM.StepSize  ASMProperties=struct('Name','BASIC_ROADS','Version','12.0','Library','ASM_Environment_lib')  ASMInstanceName=basic_roads  ASMInstanceID=1
  Bus Creator1 : BusCreator  Inputs=4
  Bus Creator2 : BusCreator  Inputs=2
  Bus Creator3 : BusCreator  Inputs=4
  Bus Selector : BusSelector  OutputSignals=ModeSignals.Road_Mode[1NoRoad|2Straight|3Circle|4Road],MdlControl.Reset_VehicleStates[0|1],InitialVehStates.Pos_z_Vehicle_Rel_Init[m],MdlControl.Get_VehPos_Trigger[],Parameters.Curv_Road_Circle[1|m]
  Bus Selector1 : BusSelector  OutputSignals=VehicleMovement.Positions.Pos_Vehicle_CoorSys_E[x;y;z][m].Pos_x_Vehicle_CoorSys_E[m],VehicleMovement.Positions.Pos_Vehicle_CoorSys_E[x;y;z][m].Pos_y_Vehicle_CoorSys_E[m],VehicleMovement.Positions.Angle_Vehicle_CoorSys_E[x;y;z][deg].Angle_Yaw_Vehicle_CoorSys_E[deg],Tire.Pos_CP_CoorSys_E[:][x;y][m]
  Bus Selector2 : BusSelector  OutputSignals=Slope_BasicRoad[%],Slope_Lateral_BasicRoad[deg],Fric_Coeff_CP_BasicRoad[:][],Sw_Tire_Parameter_Set_CP_BasicRoad[:][1|2|3|4]
  Bus Selector3 : BusSelector  OutputSignals=Route_Id_Fellows_Ref_Scheduler[],Direction_Fellows_Ref_Scheduler[-1|1],s_Fellows_Ref_Scheduler[m],d_Fellows_Ref_Scheduler[m],LaneIdx_Fellows_Ref_Scheduler[],v_Lat_Fellows_Ref_Scheduler[m|s],ForceToRoad_Fellows_Ref_Scheduler[0|1],Flag_FellowUsed[0|1],Dist_Def_Trf[]
  Bus Selector5 : BusSelector  OutputSignals=MdlControl.RoadControl[],InitialVehStates.Pos_z_Vehicle_Rel_Init[m],InitialVehStates.Angle_Yaw_Vehicle_Rel_Init[deg],InitialVehStates.Route_Id_Init[],InitialVehStates.Route_Direction_Init[],InitialVehStates.s_Vehicle_Init[m],InitialVehStates.d_Vehicle_Init[m],InitialVehStates.LaneIdx_Vehicle_Init[],RefSignals.d_Maneuver[m],RefSignals.LaneIdx_Maneuver[],Parameters.v_Lat[m|s],ModeSignals.ForceToRoad_Mode[1Off|2On],RefSignals.Dist_Def_Maneuver[]
  Bus Selector6 : BusSelector  OutputSignals=VehicleMovement.Positions.Angle_Vehicle_CoorSys_E[x;y;z][deg].Angle_Yaw_Vehicle_CoorSys_E[deg],VehicleMovement.Positions.Pos_Vehicle_CoorSys_E[x;y;z][m].Pos_x_Vehicle_CoorSys_E[m],VehicleMovement.Positions.Pos_Vehicle_CoorSys_E[x;y;z][m].Pos_y_Vehicle_CoorSys_E[m],Tire.Pos_CP_CoorSys_E[:][x;y][m],VehicleMovement.Velocities.v_x_Vehicle[km|h]
  Bus Selector7 : BusSelector  OutputSignals=VehicleMovement.Positions.Pos_Vehicle_CoorSys_E[x;y;z][m].Pos_x_Vehicle_CoorSys_E[m],VehicleMovement.Positions.Pos_Vehicle_CoorSys_E[x;y;z][m].Pos_y_Vehicle_CoorSys_E[m],VehicleMovement.Positions.RotationMatrix_V_to_E[3x3]
  Const_4Road : Constant  Value=4
  Constant1 : Constant  Value=0
  Constant2 : Constant  Value=0
  Customize_UserSignals : Subsystem
  GPS_POSITION : ASM_Environment_lib/Environment/Road/GPS_POSITION  Tag=ASM_SUBCOMPONENT  ASMProperties=struct('Name','GPS_POSITION','Version','1.0','Library','ASM_Environment_lib')  ASMInstanceName=gps_position  ASMInstanceID=1
  LANESENSOR_DYNAMIC_OUTPUT : ASM_Environment_lib/Environment/Road/LANESENSOR_DYNAMIC_OUTPUT  Const_SensorPoints_OutputDimension=MDL.Environment.Road.LaneSensorDynamic_Output.Const_SensorPoints_OutputDimension  Const_MeasPoints_OutputDimension=MDL.Environment.Road.LaneSensorDynamic_Output.Const_MeasPoints_OutputDimension  Const_LanesLeft_OutputDimension=MDL.Environment.Road.LaneSensorDynamic_Output.Const_LanesLeft_OutputDimension  Const_LanesRight_OutputDimension=MDL.Environment.Road.LaneSensorDynamic_Output.Const_LanesRight_OutputDimension  ASMProperties=struct('Name','LANESENSOR_DYNAMIC_OUTPUT','Version','2.0','Library','ASM_Environment_lib')  ASMInstanceName=lanesensor_dynamic_output  ASMInstanceID=1
  LANESENSOR_DYNAMIC_PARAMETERS : ASM_Environment_lib/Environment/Road/LANESENSOR_DYNAMIC_PARAMETERS  Tag=ASM_SUBCOMPONENT  Sw_LaneSensor_Enable=MDL.Environment.Road.LaneSensorDynamic_Parameters.Sw_LaneSensor_Enable  Const_Dist_LaneSensor=MDL.Environment.Road.LaneSensorDynamic_Parameters.Const_Dist_LaneSensor  Sw_LaneSensor_Border_Mode=MDL.Environment.Road.LaneSensorDynamic_Parameters.Sw_LaneSensor_Border_Mode  Sw_LaneSensor_Junction_Enable=MDL.Environment.Road.LaneSensorDynamic_Parameters.Sw_LaneSensor_Junction_Enable  Const_NumLanes_Left=MDL.Environment.Road.LaneSensorDynamic_Parameters.Const_NumLanes_Left  Const_NumLanes_Right=MDL.Environment.Road.LaneSensorDynamic_Parameters.Const_NumLanes_Right  Sw_LaneSensor_MeasPoint_Enable=MDL.Environment.Road.LaneSensorDynamic_Parameters.Sw_LaneSensor_MeasPoint_Enable  Const_Pos_MeasPoint_1=MDL.Environment.Road.LaneSensorDynamic_Parameters.Const_Pos_MeasPoint_1  Const_Pos_MeasPoint_2=MDL.Environment.Road.LaneSensorDynamic_Parameters.Const_Pos_MeasPoint_2  Const_Pos_MeasPoint_3=MDL.Environment.Road.LaneSensorDynamic_Parameters.Const_Pos_MeasPoint_3  Const_Pos_MeasPoint_4=MDL.Environment.Road.LaneSensorDynamic_Parameters.Const_Pos_MeasPoint_4  ASMProperties=struct('Name','LANESENSOR_DYNAMIC_PARAMETERS','Version','1.0','Library','ASM_Environment_lib')  ASMInstanceName=lanesensor_dynamic_parameters  ASMInstanceID=1
  LaneID : Display
  Left : Display
  Left1 : Display
  Mux : Mux  Inputs=2
  NoRoad : RelationalOperator  Operator===  OutDataTypeStr=boolean  RndMeth=Nearest
  Product1 : Product  RndMeth=Zero
  Product8 : Product  RndMeth=Zero
  ROAD : ASM_Environment_lib/Environment/Road/ROAD  Tag=ASM_SUBCOMPONENT  Road_ModelDesk=MDL.Environment.Road.Road_ModelDesk  Road_2=MDL.Environment.Road.Road_2  Road_3=MDL.Environment.Road.Road_3  Road_4=MDL.Environment.Road.Road_4  Road_5=MDL.Environment.Road.Road_5  Road_6=MDL.Environment.Road.Road_6  ASMProperties=struct('Name','ROAD','Version','25.0','Library','ASM_Environment_lib')  ASMInstanceName=road  ASMInstanceID=1
  Right : Display
  Right1 : Display
  Sat_RoadMode : Saturate  UpperLimit=4  LowerLimit=1
  SignalRouting : Subsystem
  Terminator : Terminator
  distance2TargetLaneLines : Subsystem  Description=This Block was created to find out distance of car center to the lines of the next lane for the lane change maneuvour
      mask Display: image('lane_line_distance.jpg');
  ones26 : Constant  Value=ones(1,26)  OutDataTypeStr=double
  zero : Constant  Value=0
  Road_Signals : Outport
  tag scope: ASMBUS_Environment_Ambient=global, ASMBUS_Environment_BasicRoads=global, ASMBUS_Environment_Customized_UserSignals=global, ASMBUS_Environment_LaneSensor_Dynamic_Output=global, ASMBUS_Environment_LaneSensor_Dynamic_Parameters=global, ASMBUS_Environment_PosVehGPS=global, ASMBUS_Environment_StandardRoad=global
  wires:
  Bus Selector7/3 -> LANESENSOR_DYNAMIC_PARAMETERS/3  "<RotationMatrix_V_to_E[3x3]>"
  ROAD/7 -> Terminator/1
  LANESENSOR_DYNAMIC_OUTPUT/2 -> SignalRouting/11(LaneSensor_Dynamic), distance2TargetLaneLines/1(posVeh_y)
  ROAD/11 -> LANESENSOR_DYNAMIC_OUTPUT/1
  LANESENSOR_DYNAMIC_OUTPUT/1 -> [ASMBUS_Environment_LaneSensor_Dynamic_Output]
  Bus Selector7/2 -> LANESENSOR_DYNAMIC_PARAMETERS/2  "<Pos_y_Vehicle_CoorSys_E[m]>"
  Bus Selector7/1 -> LANESENSOR_DYNAMIC_PARAMETERS/1  "<Pos_x_Vehicle_CoorSys_E[m]>"
  LANESENSOR_DYNAMIC_PARAMETERS/1 -> [ASMBUS_Environment_LaneSensor_Dynamic_Parameters]
  BASIC_ROADS/5 -> Bus Creator1/4
  s_Preview[m]/1 -> Mux/2, BASIC_ROADS/6
  ROAD/5 -> Bus Creator3/4
  Mux/1 -> ROAD/15
  Product8/1 -> ROAD/11
  Product1/1 -> ROAD/10
  LANESENSOR_DYNAMIC_PARAMETERS/8 -> ROAD/37
  LANESENSOR_DYNAMIC_PARAMETERS/7 -> ROAD/36
  LANESENSOR_DYNAMIC_PARAMETERS/6 -> ROAD/35
  LANESENSOR_DYNAMIC_PARAMETERS/5 -> ROAD/34
  LANESENSOR_DYNAMIC_PARAMETERS/4 -> ROAD/33
  LANESENSOR_DYNAMIC_PARAMETERS/2 -> ROAD/31
  LANESENSOR_DYNAMIC_PARAMETERS/3 -> ROAD/32
  ROAD/10 -> SignalRouting/7(TrafficObject_Data)
  Bus Selector5/13 -> ROAD/14  "<Dist_Def_Maneuver[]>"
  Bus Selector5/4 -> ROAD/5  "<Route_Id_Init[]>"
  Bus Selector5/5 -> ROAD/6  "<Route_Direction_Init[]>"
  Bus Selector3/9 -> ROAD/30  "<Dist_Def_Trf[]>"
  Bus Selector3/1 -> ROAD/22  "<Route_Id_Fellows_Ref_Scheduler[]>"
  Bus Selector3/2 -> ROAD/23  "<Direction_Fellows_Ref_Scheduler[-1|1]>"
  AMBIENT/1 -> [ASMBUS_Environment_Ambient]
  Traffic_Signals/1 -> Bus Selector3/1
  [TAG_Sw_BasicRoad] -> Bus Selector2/1
  Sat_RoadMode/1 -> NoRoad/1
  Bus Selector/1 -> Sat_RoadMode/1, BASIC_ROADS/1  "<Road_Mode[1NoRoad|2Straight|3Circle|4Road]>"
  VehicleDynamics_Signals/1 -> Bus Selector1/1, Bus Selector6/1, Bus Selector7/1
  Maneuver_Signals/1 -> Bus Selector5/1, Bus Selector/1
  SignalRouting/1(Road) -> Road_Signals/1
  BASIC_ROADS/1 -> [ASMBUS_Environment_BasicRoads]
  [TAG_Sw_RoadSelect] -> ROAD/1
  Bus Selector5/1 -> ROAD/2  "<RoadControl[]>"
  Bus Selector5/6 -> ROAD/7  "<s_Vehicle_Init[m]>"
  Bus Selector5/8 -> ROAD/9  "<LaneIdx_Vehicle_Init[]>"
  Bus Selector5/11 -> ROAD/12  "<v_Lat[m|s]>"
  Bus Selector5/12 -> ROAD/13  "<ForceToRoad_Mode[1Off|2On]>"
  zero/1 -> Mux/1
  Bus Selector1/1 -> ROAD/16, GPS_POSITION/2  "<Pos_x_Vehicle_CoorSys_E[m]>"
  Bus Selector1/2 -> ROAD/17, distance2TargetLaneLines/2(Input), GPS_POSITION/3  "<Pos_y_Vehicle_CoorSys_E[m]>"
  Bus Selector1/3 -> ROAD/18  "<Angle_Yaw_Vehicle_CoorSys_E[deg]>"
  Bus Selector1/4 -> ROAD/19  "<Pos_CP_CoorSys_E[:][x;y][m]>"
  Bus Selector3/3 -> ROAD/24  "<s_Fellows_Ref_Scheduler[m]>"
  Bus Selector3/4 -> ROAD/25  "<d_Fellows_Ref_Scheduler[m]>"
  Bus Selector3/5 -> ROAD/26  "<LaneIdx_Fellows_Ref_Scheduler[]>"
  Bus Selector3/6 -> ROAD/27  "<v_Lat_Fellows_Ref_Scheduler[m|s]>"
  Bus Selector3/7 -> ROAD/28  "<ForceToRoad_Fellows_Ref_Scheduler[0|1]>"
  Const_4Road/1 -> NoRoad/2
  NoRoad/1 -> SignalRouting/1(SwitchRoad[0BasicRoad|1StandardRoad]), ASMSignalCollector/1(SwitchRoad[0BasicRoad|1StandardRoad])
  ROAD/1 -> [ASMBUS_Environment_StandardRoad]
  ROAD/6 -> SignalRouting/4(Info)
  ROAD/8 -> SignalRouting/5(TrafficFellows)
  ROAD/9 -> Customize_UserSignals/1(UserSignals_In), SignalRouting/6(UserSignals)
  AMBIENT/2 -> Bus Creator2/1  "T_Ambient[degC]"
  AMBIENT/3 -> Bus Creator2/2  "p_Ambient[Pa]"
  GPS_POSITION/2 -> SignalRouting/9(Pos_Vehicle_GPS[Long;Lat][deg])
  Constant1/1 -> ROAD/20
  Constant2/1 -> ROAD/21
  Bus Selector5/10 -> Product8/2  "<LaneIdx_Maneuver[]>"
  ones26/1 -> Product8/1, Product1/2
  Bus Selector/2 -> BASIC_ROADS/2  "<Reset_VehicleStates[0|1]>"
  Bus Selector/3 -> BASIC_ROADS/3  "<Pos_z_Vehicle_Rel_Init[m]>"
  Bus Selector/4 -> BASIC_ROADS/4  "<Get_VehPos_Trigger[]>"
  Bus Selector/5 -> BASIC_ROADS/5  "<Curv_Road_Circle[1|m]>"
  Bus Selector6/1 -> BASIC_ROADS/7  "<Angle_Yaw_Vehicle_CoorSys_E[deg]>"
  Bus Selector6/2 -> BASIC_ROADS/8  "<Pos_x_Vehicle_CoorSys_E[m]>"
  Bus Selector6/3 -> BASIC_ROADS/9  "<Pos_y_Vehicle_CoorSys_E[m]>"
  Bus Selector6/4 -> BASIC_ROADS/10  "<Pos_CP_CoorSys_E[:][x;y][m]>"
  Bus Selector6/5 -> BASIC_ROADS/11  "<v_x_Vehicle[km|h]>"
  Bus Selector2/1 -> BASIC_ROADS/12  "<Slope_BasicRoad[%]>"
  Bus Selector2/2 -> BASIC_ROADS/13  "<Slope_Lateral_BasicRoad[deg]>"
  Bus Selector2/3 -> BASIC_ROADS/14  "<Fric_Coeff_CP_BasicRoad[:][]>"
  Bus Selector2/4 -> BASIC_ROADS/15  "<Sw_Tire_Parameter_Set_CP_BasicRoad[:][1|2|3|4]>"
  BASIC_ROADS/2 -> Bus Creator1/1
  BASIC_ROADS/3 -> Bus Creator1/2
  BASIC_ROADS/4 -> Bus Creator1/3
  ROAD/2 -> Bus Creator3/1
  ROAD/3 -> Bus Creator3/2
  ROAD/4 -> Bus Creator3/3
  Bus Creator1/1 -> SignalRouting/2(BasicRoad)
  Bus Creator3/1 -> SignalRouting/3(StandardRoad)
  Bus Creator2/1 -> SignalRouting/10(Ambient)  "Ambient"
  Customize_UserSignals/2(UserSignals_Customized) -> SignalRouting/8(Customized_UserSignals), GPS_POSITION/1
  Customize_UserSignals/1(ASMSignalBus) -> [ASMBUS_Environment_Customized_UserSignals]
  GPS_POSITION/1 -> [ASMBUS_Environment_PosVehGPS]
  Bus Selector5/7 -> ROAD/8  "<d_Vehicle_Init[m]>"
  Bus Selector5/9 -> Product1/1  "<d_Maneuver[m]>"
  Bus Selector3/8 -> ROAD/29  "<Flag_FellowUsed[0|1]>"
  Bus Selector5/2 -> ROAD/3  "<Pos_z_Vehicle_Rel_Init[m]>"
  Bus Selector5/3 -> ROAD/4  "<Angle_Yaw_Vehicle_Rel_Init[deg]>"
  distance2TargetLaneLines/1(LeftLineDistance) -> Left/1
  distance2TargetLaneLines/2(RightLineDistance) -> Right/1
  distance2TargetLaneLines/3(Right) -> Left1/1
  distance2TargetLaneLines/4(Left) -> Right1/1
  distance2TargetLaneLines/5(Lane_ID) -> LaneID/1

== system ASM_Traffic_V2X_Complete_Model_2/MDL/Environment/Traffic ==
  Road_Signals : Inport
  Maneuver_Signals : Inport  Port=2
  VehicleDynamics_Signals : Inport  Port=3
  ASMSignalCollector : Subsystem
  Bus Creator1 : BusCreator  Inputs=3
  FellowMovement : Subsystem
  ObjectParameters : Subsystem
  Sensors : Subsystem
  Traffic_Signals_toRoad : Outport
  Traffic_Signals : Outport  Port=2
  wires:
  ObjectParameters/1(Objects_Signals) -> FellowMovement/4(Objects_Signals), Sensors/3(Objects_Signals), Bus Creator1/3  "Objects_Signals"
  FellowMovement/2(Fellows_Signals) -> Sensors/1(Fellows_Signals), Bus Creator1/1
  Sensors/1(Sensor_Signals) -> Bus Creator1/2
  FellowMovement/1(Traffic_Signals_toRoad) -> Traffic_Signals_toRoad/1
  Bus Creator1/1 -> Traffic_Signals/1  "Traffic"
  VehicleDynamics_Signals/1 -> Sensors/2(VehicleDynamics_Signals), FellowMovement/3(VehicleDynamics_Signals)
  Maneuver_Signals/1 -> Sensors/5(Maneuver_Signals), ObjectParameters/1(Maneuver_Signals), FellowMovement/2(Maneuver_Signals)
  Road_Signals/1 -> Sensors/4(Road_Signals), FellowMovement/1(Road_Signals)

== system ASM_Traffic_V2X_Complete_Model_2/MDL/MDL_In/Ctrl_CentralDiff[%] ==
  SoftECU : Inport
  RealECU : Inport  Port=2
  Const_Ctrl_CentralDiff[%] : Constant  Value=0
  MultiPortSwitch : MultiPortSwitch  SaturateOnIntegerOverflow=on  InputSameDT=on
  Sw_Ctrl_CentralDiff[1SoftECU|2RealECU|3Const] : Constant  Value=CPT.MDL_SW.Sw_Ctrl_CentralDiff.v
  Ctrl_CentralDiff[%] : Outport
  wires:
  MultiPortSwitch/1 -> Ctrl_CentralDiff[%]/1
  Const_Ctrl_CentralDiff[%]/1 -> MultiPortSwitch/4
  RealECU/1 -> MultiPortSwitch/3
  SoftECU/1 -> MultiPortSwitch/2
  Sw_Ctrl_CentralDiff[1SoftECU|2RealECU|3Const]/1 -> MultiPortSwitch/1
